simulink model "BEV_R2021b"  (R2022a)
settings: Solver=ode4  StartTime=0.0  StopTime=4012  FixedStep=0.01  RelTol=1e-3
undefined symbols (not defined in the file or in its folder): A, C0, Cd, g, i, N, n, r, SOCint, Vehicle_Mass
libraries: autolibshared x2, autolibshareddiff x1
(part 1 of 2)
settings Model: Creator=atong  LastModifiedBy=39829
settings DebuggingCC: UnconnectedInputMsg=warning  UnconnectedOutputMsg=warning  UnconnectedLineMsg=warning
settings RTWCC: DLArmComputeVersion=19.05

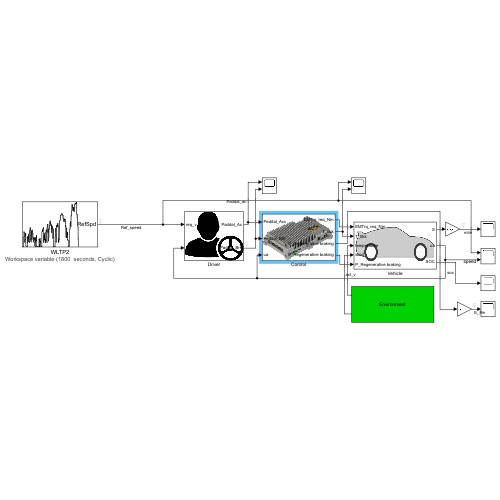
[thumbnail: Simulink's stored preview of the top-level diagram]
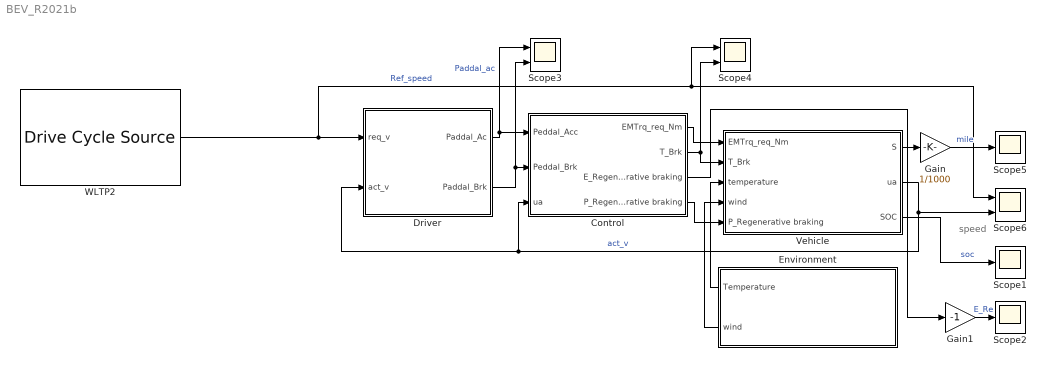
== system BEV_R2021b ==
  note: speed
  Control : Subsystem
      mask Display: image('$imagefile'); % 使用工具条上的 "编辑图像" 进行更改。
  Driver : Subsystem
      mask Display: image('$imagefile'); % 使用工具条上的 "编辑图像" 进行更改。
  Environment : Subsystem
      mask Display: disp(getString(message('autoblks:autoblkVehMask:environ')))
  Gain : Gain  Gain=1/1000
  Gain1 : Gain  Gain=-1
  Scope1 : Scope
  Scope2 : Scope
  Scope3 : Scope  NumInputPorts=2
  Scope4 : Scope  NumInputPorts=2
  Scope5 : Scope
  Scope6 : Scope  NumInputPorts=2
  Vehicle : Subsystem
      mask Display: image('$imagefile'); % 使用工具条上的 "编辑图像" 进行更改。
  WLTP2 : autolibshared/Drive Cycle Source  cycleVar=Workspace variable  wsVar=sch_cycle  fileVar=cycleFTP75.mat  tfinal="1800  seconds, Cyclic"  cycleRepeat=on  outAccPort=off  outGearPort=off  gearList=No gear data  t_wot1=5  xdot_woto=0  xdot_wot1=30  t_wot2=20  xdot_wot2=0  t_wotend=30  srcUnit=m/s  outUnit=m/s  srcAccUnit=m/s/s  outAccUnit=m/s^2  dt=0  aMode=1  faultOption=off  velBnd=2  velBndUnit=mph  inUnit=m/s  timeBnd=1  failOption=off  stopSim=off  maxFaultCnt=10  maxFaultTime=2  maxTotFaultTime=15  traceOption=off  dtTrace=1  traceWindow=10  lastDCname=Custom Data Set  lastOutUnit=mph  lastDT=0  lastTB=1  lastSB=2  forceCalcBound=off
      settings: SourceProductBaseCode=PW,DR,MT,VE
  wires:
  Driver/1(Paddal_Ac) -> Scope3/1, Control/1(Peddal_Acc)  "Paddal_ac"
  Driver/2(Paddal_Brk) -> Scope3/2, Control/2(Peddal_Brk)
  Control/2(T_Brk) -> Vehicle/2(T_Brk), Scope4/2
  Vehicle/2(ua) -> Scope6/2, Control/3(ua), Driver/2(act_v)  "act_v"
  Vehicle/1(S) -> Gain/1
  Vehicle/3(SOC) -> Scope1/1  "soc"
  WLTP2/1 -> Scope6/1, Scope4/1, Driver/1(req_v)  "Ref_speed"
  Gain/1 -> Scope5/1  "mile"
  Control/1(EMTrq_req_Nm) -> Vehicle/1(EMTrq_req_Nm)
  Environment/1(Temperature) -> Vehicle/3(temperature)
  Environment/2(wind) -> Vehicle/4(wind)
  Control/3(E_Regenerative braking) -> Gain1/1
  Control/4(P_Regenerative braking) -> Vehicle/5(P_Regenerative braking)
  Gain1/1 -> Scope2/1  "E_Re"

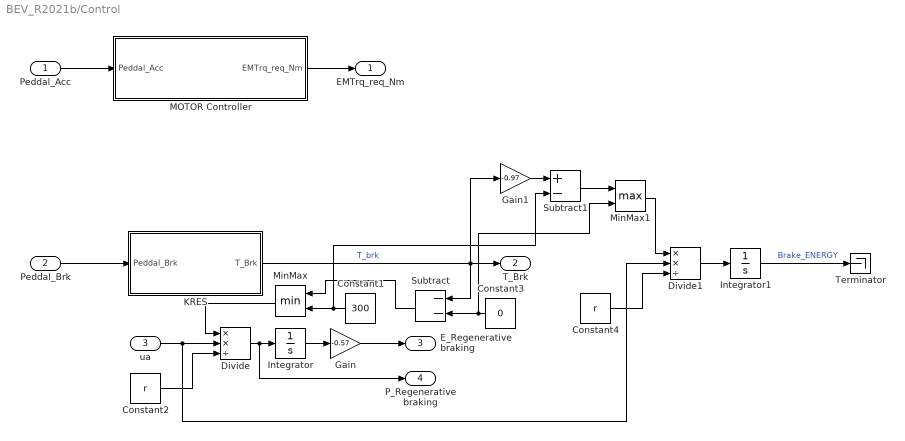
== system BEV_R2021b/Control ==
  Peddal_Acc : Inport
  Peddal_Brk : Inport  Port=2
  ua : Inport  Port=3
  Constant1 : Constant  Value=300
  Constant2 : Constant  Value=r
  Constant3 : Constant  Value=0
  Constant4 : Constant  Value=r
  Divide : Product  Inputs=**/
  Divide1 : Product  Inputs=**/
  Gain : Gain  Gain=-0.57
  Gain1 : Gain  Gain=-0.97
  Integrator : Integrator
  Integrator1 : Integrator
  KRES : Subsystem
  MOTOR Controller : Subsystem
  MinMax : MinMax  Inputs=2
  MinMax1 : MinMax  Function=max  Inputs=2
  Subtract : Sum  Inputs=--
  Subtract1 : Sum  Inputs=+-
  Terminator : Terminator
  EMTrq_req_Nm : Outport
  T_Brk : Outport  Port=2
  E_Regenerative braking : Outport  Port=3
  P_Regenerative braking : Outport  Port=4
  wires:
  Peddal_Brk/1 -> KRES/1(Peddal_Brk)
  KRES/1(T_Brk) -> Gain1/1, Subtract/1, T_Brk/1  "T_brk"
  Peddal_Acc/1 -> MOTOR Controller/1(Peddal_Acc)
  MOTOR Controller/1(EMTrq_req_Nm) -> EMTrq_req_Nm/1
  Constant2/1 -> Divide/3
  Divide/1 -> P_Regenerative braking/1, Integrator/1
  Integrator/1 -> Gain/1
  Gain/1 -> E_Regenerative braking/1
  MinMax/1 -> Divide/1
  Constant1/1 -> Subtract1/2, MinMax/2
  Subtract/1 -> MinMax/1
  Constant3/1 -> MinMax1/2, Subtract/2
  ua/1 -> Divide1/2, Divide/2
  Constant4/1 -> Divide1/3
  Integrator1/1 -> Terminator/1  "Brake_ENERGY"
  MinMax1/1 -> Divide1/1
  Gain1/1 -> Subtract1/1
  Subtract1/1 -> MinMax1/1
  Divide1/1 -> Integrator1/1

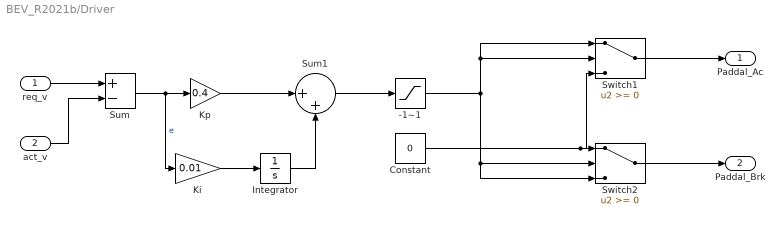
== system BEV_R2021b/Driver ==
  req_v : Inport
  act_v : Inport  Port=2
  -1~1 : Saturate  UpperLimit=1  LowerLimit=-1
  Constant : Constant  Value=0
  Integrator : Integrator
  Ki : Gain  Gain=0.01
  Kp : Gain  Gain=0.4
  Sum : Sum  Inputs=+-
  Sum1 : Sum  Inputs=|++
  Switch1 : Switch  SaturateOnIntegerOverflow=off  InputSameDT=off
  Switch2 : Switch  SaturateOnIntegerOverflow=off  InputSameDT=off
  Paddal_Ac : Outport
  Paddal_Brk : Outport  Port=2
  wires:
  Constant/1 -> Switch1/3, Switch2/1
  Switch2/1 -> Paddal_Brk/1
  Switch1/1 -> Paddal_Ac/1
  -1~1/1 -> Switch2/3, Switch2/2, Switch1/1, Switch1/2
  Integrator/1 -> Sum1/2
  Ki/1 -> Integrator/1
  Sum1/1 -> -1~1/1
  Kp/1 -> Sum1/1
  req_v/1 -> Sum/1
  act_v/1 -> Sum/2
  Sum/1 -> Ki/1, Kp/1  "e"

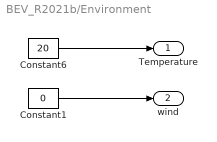
== system BEV_R2021b/Environment ==
  Constant1 : Constant  Value=0
  Constant6 : Constant  Value=20
  Temperature : Outport  VectorParamsAs1DForOutWhenUnconnected=off
  wind : Outport  Port=2  VectorParamsAs1DForOutWhenUnconnected=off
  wires:
  Constant6/1 -> Temperature/1
  Constant1/1 -> wind/1

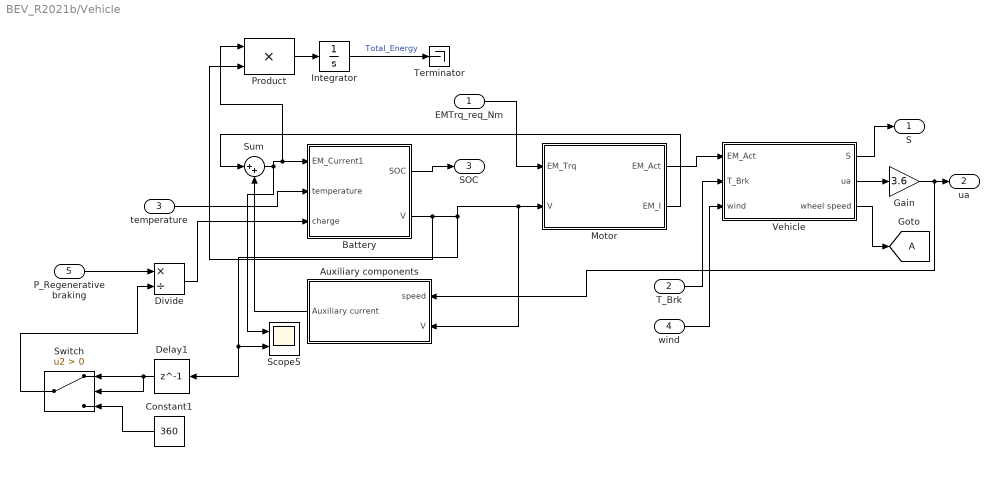
== system BEV_R2021b/Vehicle ==
  EMTrq_req_Nm : Inport
  T_Brk : Inport  Port=2
  temperature : Inport  Port=3
  wind : Inport  Port=4
  P_Regenerative braking : Inport  Port=5
  Auxiliary components : Subsystem
  Battery : Subsystem
      mask Display: image('$imagefile'); % 使用工具条上的 "编辑图像" 进行更改。
  Constant1 : Constant  Value=360
  Delay1 : Delay  DelayLength=1  InitialCondition=0
  Divide : Product  Inputs=*/
  Gain : Gain  Gain=3.6
  Goto : Goto  TagVisibility=global
  Integrator : Integrator
  Motor : Subsystem
      mask Display: image('$imagefile'); % 使用工具条上的 "编辑图像" 进行更改。
  Product : Product
  Scope5 : Scope  NumInputPorts=2
  Sum : Sum  Inputs=|++
  Switch : Switch  Criteria=u2 > Threshold  SaturateOnIntegerOverflow=off  InputSameDT=off
  Terminator : Terminator
  Vehicle : Subsystem
      mask Display: image('$imagefile'); % 使用工具条上的 "编辑图像" 进行更改。
  S : Outport
  ua : Outport  Port=2
  SOC : Outport  Port=3
  wires:
  EMTrq_req_Nm/1 -> Motor/1(EM_Trq)
  Motor/1(EM_Act) -> Vehicle/1(EM_Act)
  T_Brk/1 -> Vehicle/2(T_Brk)
  Vehicle/1(S) -> S/1
  Battery/1(SOC) -> SOC/1
  Vehicle/3(wheel speed) -> Goto/1
  temperature/1 -> Battery/2(temperature)
  wind/1 -> Vehicle/3(wind)
  Gain/1 -> Auxiliary components/1(speed), ua/1
  Vehicle/2(ua) -> Gain/1
  Auxiliary components/1(Auxiliary current) -> Sum/2
  Motor/2(EM_I) -> Sum/1
  Sum/1 -> Product/1, Battery/1(EM_Current1), Scope5/1
  Divide/1 -> Battery/3(charge)
  P_Regenerative braking/1 -> Divide/1
  Switch/1 -> Divide/2
  Constant1/1 -> Switch/3
  Battery/2(V) -> Product/2, Auxiliary components/2(V), Motor/2(V), Delay1/1, Scope5/2
  Delay1/1 -> Switch/2, Switch/1
  Product/1 -> Integrator/1
  Integrator/1 -> Terminator/1  "Total_Energy"

== system BEV_R2021b/Control/KRES ==
  Peddal_Brk : Inport
  Constant : Constant  Value=800
  Product : Product
  T_Brk : Outport
  wires:
  Product/1 -> T_Brk/1
  Peddal_Brk/1 -> Product/1
  Constant/1 -> Product/2

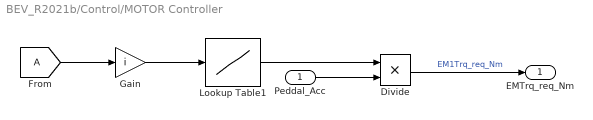
== system BEV_R2021b/Control/MOTOR Controller ==
  Peddal_Acc : Inport
  Divide : Product  Inputs=**
  From : From  TagVisibility=global
  Gain : Gain  Gain=i
  Lookup Table1 : Lookup  InputValues=[500,1000,2000,3000,4000,5000,6000,7000,10000,12000]  Table=[131,130,129,128,81,65,54,46,40,38]  SaturateOnIntegerOverflow=off
  EMTrq_req_Nm : Outport
  wires:
  Gain/1 -> Lookup Table1/1
  From/1 -> Gain/1
  Divide/1 -> EMTrq_req_Nm/1  "EM1Trq_req_Nm"
  Lookup Table1/1 -> Divide/1
  Peddal_Acc/1 -> Divide/2

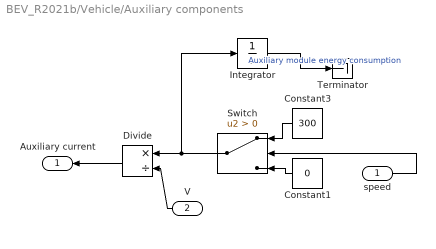
== system BEV_R2021b/Vehicle/Auxiliary components ==
  speed : Inport
  V : Inport  Port=2
  Constant1 : Constant  Value=0
  Constant3 : Constant  Value=300
  Divide : Product  Inputs=*/
  Integrator : Integrator
  Switch : Switch  Criteria=u2 > Threshold  SaturateOnIntegerOverflow=off  InputSameDT=off
  Terminator : Terminator
  Auxiliary current : Outport
  wires:
  Constant1/1 -> Switch/3
  Constant3/1 -> Switch/1
  Divide/1 -> Auxiliary current/1
  V/1 -> Divide/2
  speed/1 -> Switch/2
  Switch/1 -> Integrator/1, Divide/1
  Integrator/1 -> Terminator/1  "Auxiliary module energy consumption"

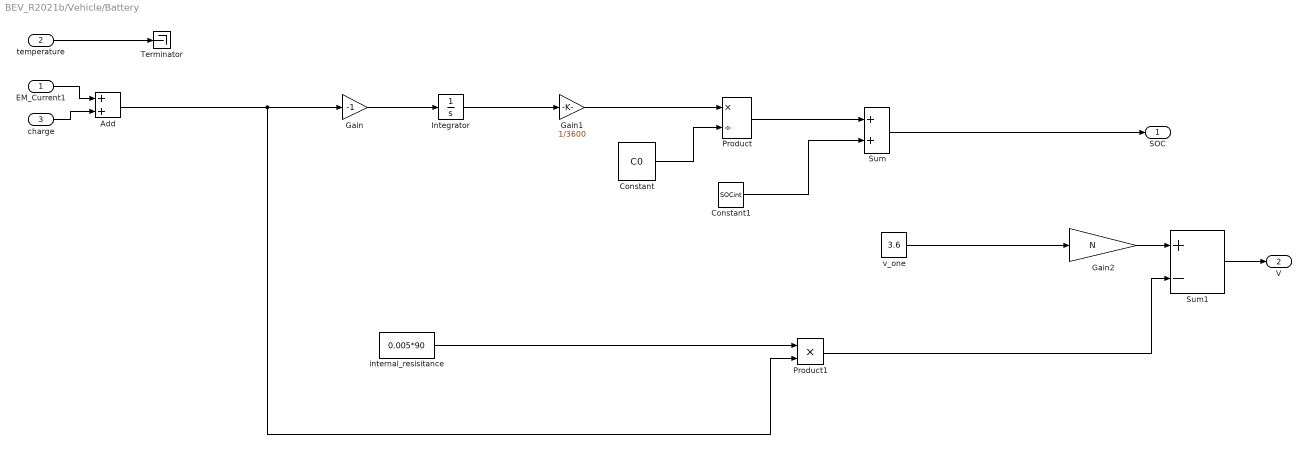
== system BEV_R2021b/Vehicle/Battery ==
  EM_Current1 : Inport
  temperature : Inport  Port=2
  charge : Inport  Port=3
  Add : Sum
  Constant : Constant  Value=C0
  Constant1 : Constant  Value=SOCint
  Gain : Gain  Gain=-1
  Gain1 : Gain  Gain=1/3600
  Gain2 : Gain  Gain=N
  Integrator : Integrator
  Product : Product  Inputs=*/
  Product1 : Product
  Sum : Sum
  Sum1 : Sum  Inputs=+-
  Terminator : Terminator
  internal_resisitance : Constant  Value=0.005*90
  v_one : Constant  Value=3.6
  SOC : Outport
  V : Outport  Port=2
  wires:
  Add/1 -> Product1/2, Gain/1
  Gain/1 -> Integrator/1
  Integrator/1 -> Gain1/1
  Gain1/1 -> Product/1
  Constant/1 -> Product/2
  Product/1 -> Sum/1
  Constant1/1 -> Sum/2
  Sum/1 -> SOC/1
  v_one/1 -> Gain2/1
  Gain2/1 -> Sum1/1
  Product1/1 -> Sum1/2
  Sum1/1 -> V/1
  internal_resisitance/1 -> Product1/1
  temperature/1 -> Terminator/1
  charge/1 -> Add/2
  EM_Current1/1 -> Add/1

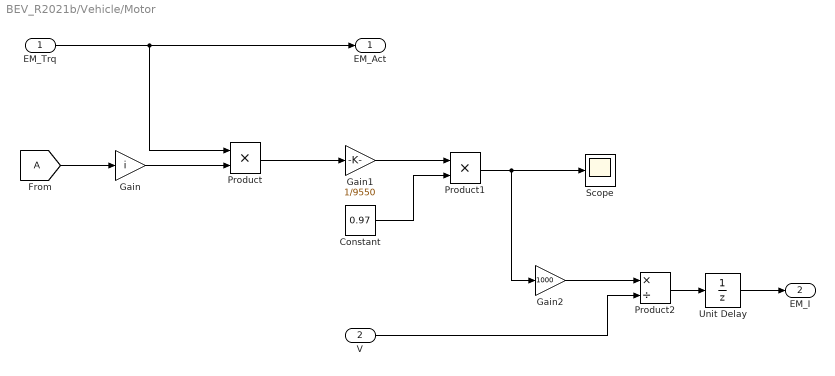
== system BEV_R2021b/Vehicle/Motor ==
  EM_Trq : Inport
  V : Inport  Port=2
  Constant : Constant  Value=0.97
  From : From  TagVisibility=global
  Gain : Gain  Gain=i
  Gain1 : Gain  Gain=1/9550
  Gain2 : Gain  Gain=1000
  Product : Product
  Product1 : Product
  Product2 : Product  Inputs=*/
  Scope : Scope
  Unit Delay : UnitDelay  SampleTime=-1  HasFrameUpgradeWarning=on
  EM_Act : Outport
  EM_I : Outport  Port=2
  wires:
  EM_Trq/1 -> EM_Act/1, Product/1
  From/1 -> Gain/1
  Gain/1 -> Product/2
  Product/1 -> Gain1/1
  Gain1/1 -> Product1/1
  Constant/1 -> Product1/2
  Product1/1 -> Scope/1, Gain2/1
  Gain2/1 -> Product2/1
  V/1 -> Product2/2
  Product2/1 -> Unit Delay/1
  Unit Delay/1 -> EM_I/1
